simulink model "ScreenControl"  (R2023a)
settings: Solver=FixedStepAuto  StartTime=0.0  StopTime=10.0  RelTol=1e-3
undefined symbols (not defined in the file or in its folder): Display1stGear, Display2ndGear, Display3rdGear, Display4thGear, Display5thGear, Display6thGear, Display7thGear, Display8thGear, Display9thGear, DisplayNGear, DisplayRGear
settings Model: Creator=Carlos  LastModifiedBy=Carlos
settings OptimizationCC: DefaultParameterBehavior=Inlined  OptimizeBlockIOStorage=off  BufferReuse=off  ReuseModelBlockBuffer=off  GlobalBufferReuse=off  ExpressionFolding=off  EnableMemcpy=off  PassReuseOutputArgsAs=Individual arguments  LocalBlockOutputs=off  ZeroExternalMemoryAtStartup=off  ZeroInternalMemoryAtStartup=off  OptimizeDataStoreBuffers=off  BusAssignmentInplaceUpdate=off  OptimizationLevel=level0  OptimizationCustomize=off  EfficientTunableParamExpr=on
settings DebuggingCC: ParameterTunabilityLossMsg=error
settings HardwareCC: ProdBitPerInt=16  ProdBitPerPointer=16  ProdBitPerSizeT=16  ProdBitPerPtrDiffT=16  ProdLargestAtomicFloat=None  ProdWordSize=8  ProdHWDeviceType=Atmel->AVR
settings SFSimCC: MATLABDynamicMemAlloc=off
settings RTWCC: Description=Embedded Coder  SystemTargetFile=ert.tlc  TemplateMakefile=ert_default_tmf  TargetLang=C++
settings CodeAppCC: ForceParamTrailComments=on  IgnoreCustomStorageClasses=off  OperatorAnnotations=on  SimulinkDataObjDesc=on  SFDataObjDesc=on  InsertBlockDesc=on
settings ERTTargetCC: TargetLangStandard=C++11 (ISO)  GenerateSampleERTMain=on  CodeInterfacePackaging=C++ class  InlinedParameterPlacement=NonHierarchical  RootIOFormat=Structure reference  ERTCustomFileTemplate=example_file_process.tlc

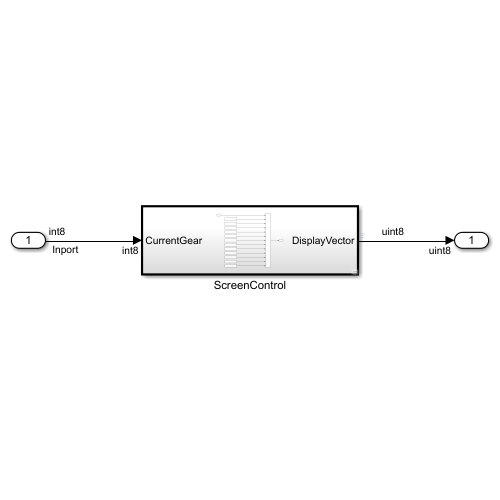
[thumbnail: Simulink's stored preview of the top-level diagram]
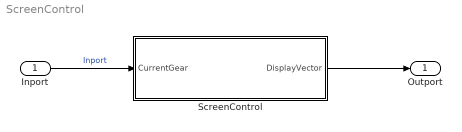
== system ScreenControl ==
  Inport : Inport
  ScreenControl : Subsystem  TreatAsAtomicUnit=on
  Outport : Outport  OutDataTypeStr=uint8
  wires:
  Inport/1 -> ScreenControl/1(CurrentGear)  "Inport"
  ScreenControl/1(DisplayVector) -> Outport/1

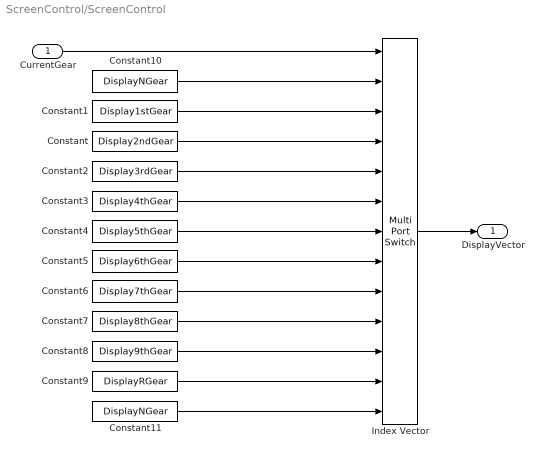
== system ScreenControl/ScreenControl ==
  CurrentGear : Inport  OutDataTypeStr=int8
  Constant : Constant  Value=Display2ndGear
  Constant1 : Constant  Value=Display1stGear
  Constant10 : Constant  Value=DisplayNGear
  Constant11 : Constant  Value=DisplayNGear
  Constant2 : Constant  Value=Display3rdGear
  Constant3 : Constant  Value=Display4thGear
  Constant4 : Constant  Value=Display5thGear
  Constant5 : Constant  Value=Display6thGear
  Constant6 : Constant  Value=Display7thGear
  Constant7 : Constant  Value=Display8thGear
  Constant8 : Constant  Value=Display9thGear
  Constant9 : Constant  Value=DisplayRGear
  Index Vector : MultiPortSwitch  DataPortOrder=Specify indices  Inputs=4  DataPortIndices={0,1,2,3,4,5,6,7,8,9,-1}  DataPortForDefault=Additional data port  DiagnosticForDefault=None  OutDataTypeStr=uint8  SaturateOnIntegerOverflow=off
  DisplayVector : Outport
  wires:
  Constant11/1 -> Index Vector/13
  Constant4/1 -> Index Vector/7
  Constant5/1 -> Index Vector/8
  Constant9/1 -> Index Vector/12
  Constant2/1 -> Index Vector/5
  Constant10/1 -> Index Vector/2
  Constant7/1 -> Index Vector/10
  Index Vector/1 -> DisplayVector/1
  Constant3/1 -> Index Vector/6
  Constant8/1 -> Index Vector/11
  Constant1/1 -> Index Vector/3
  Constant/1 -> Index Vector/4
  Constant6/1 -> Index Vector/9
  CurrentGear/1 -> Index Vector/1
